simulink model "Model"  (Simulink 9.1)
settings: Solver=VariableStepAuto  StartTime=0.0  StopTime=10.0  RelTol=1e-3
libraries: ExampleToolbox x1
settings Model: SuppressorTable=22 serialization::archive 11 0 6 0 0 0 1 0  Creator=dferigo  LastModifiedBy=dferigo
settings DataIOCC: SaveFormat=Dataset
settings OptimizationCC: LifeSpan=auto
settings DebuggingCC: UnderspecifiedInitializationDetection=Simplified  MergeDetectMultiDrivingBlocksExec=error  SFUnexpectedBacktrackingDiag=error  SFNoUnconditionalDefaultTransitionDiag=error  SFExecutionAtInitializationDiag=warning
settings HardwareCC: ProdBitPerPointer=64  ProdBitPerSizeT=64  ProdBitPerPtrDiffT=64  ProdLargestAtomicFloat=Float  ProdIntDivRoundTo=Zero  ProdEndianess=LittleEndian  ProdWordSize=64  ProdHWDeviceType=Intel->x86-64 (Windows64)
settings ModelReferenceCC: PropagateSignalLabelsOutOfModel=on
settings CodeAppCC: StateflowObjectComments=off
settings GRTTargetCC: TargetLangStandard=C99 (ISO)  CombineOutputUpdateFcns=on  GRTInterface=off
settings ConfigComp: CovMetricSettings=dwe  CovHtmlReporting=off  CovSaveCumulativeToWorkspaceVar=off  CovSaveSingleToWorkspaceVar=off  CovExternalEMLEnable=on

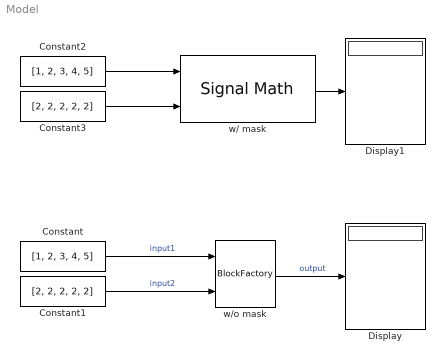
== system Model ==
  Constant : Constant  Value=[1, 2, 3, 4, 5]
  Constant1 : Constant  Value=[2, 2, 2, 2, 2]
  Constant2 : Constant  Value=[1, 2, 3, 4, 5]
  Constant3 : Constant  Value=[2, 2, 2, 2, 2]
  Display : Display
  Display1 : Display
  w/ mask : ExampleToolbox/Signal Math  operation=Multiplication
      settings: SourceProductName=Example Toolbox
  w/o mask : S-Function  FunctionName=BlockFactory  Parameters='SignalMath','ExampleToolbox','Addition'  SFunctionDeploymentMode=off  EnableBusSupport=off
  wires:
  Constant/1 -> w/o mask/1  "input1"
  Constant1/1 -> w/o mask/2  "input2"
  w/o mask/1 -> Display/1  "output"
  Constant2/1 -> w/ mask/1
  Constant3/1 -> w/ mask/2
  w/ mask/1 -> Display1/1
